simulink model "DDR_KinematicModel"  (R2019b)
settings: Solver=FixedStepAuto  StartTime=0.0  StopTime=10  FixedStep=0.001  RelTol=1e-3
undefined symbols (not defined in the file): a, phi_init, v0, x_init, xi, y_init
libraries: simulink x1
settings Model: Creator=DanielleNasrallah  LastModifiedBy=kerrm
settings DataIOCC: ReturnWorkspaceOutputs=off

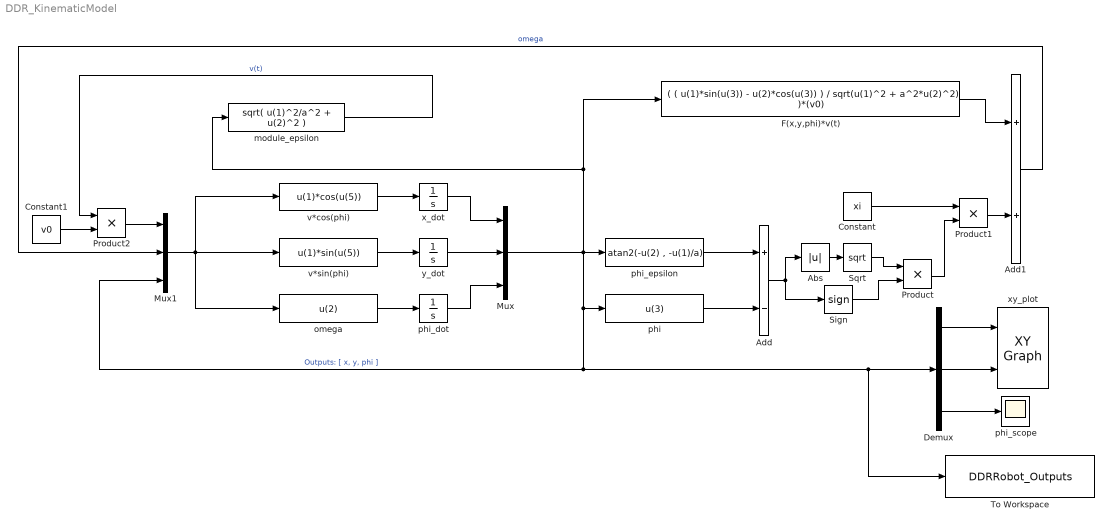
== system DDR_KinematicModel ==
  Abs : Abs
  Add : Sum  Inputs=+-
  Add1 : Sum
  Constant : Constant  Value=xi
  Constant1 : Constant  Value=v0
  Demux : Demux  Outputs=3
  F(x,y,phi)*v(t) : Fcn  Expr=( ( u(1)*sin(u(3)) - u(2)*cos(u(3)) ) / sqrt(u(1)^2 + a^2*u(2)^2) )*(v0)
  Mux : Mux  Inputs=3
  Mux1 : Mux  Inputs=3
  Product : Product
  Product1 : Product
  Product2 : Product
  Sign : Signum
  Sqrt : Sqrt  SaturateOnIntegerOverflow=on
  To Workspace : ToWorkspace  VariableName=DDRRobot_Outputs  SampleTime=-1
      settings: Save2DSignal=2-D array (concatenate along first dimension)
  "module_epsilon " : Fcn  Expr=sqrt( u(1)^2/a^2 + u(2)^2 )
  "omega " : Fcn  Expr=u(2)
  phi : Fcn  Expr=u(3)
  phi_dot : Integrator  InitialCondition=phi_init
  phi_epsilon : Fcn  Expr=atan2(-u(2) , -u(1)/a)
  phi_scope : Scope
  v*cos(phi) : Fcn  Expr=u(1)*cos(u(5))
  v*sin(phi) : Fcn  Expr=u(1)*sin(u(5))
  x_dot : Integrator  InitialCondition=x_init
  xy_plot : simulink/Sinks/XY Graph  xmin=-5  xmax=5  ymin=-5  ymax=5  st=-1
  y_dot : Integrator  InitialCondition=y_init
  wires:
  y_dot/1 -> Mux/2
  x_dot/1 -> Mux/1
  phi_dot/1 -> Mux/3
  Mux1/1 -> v*cos(phi)/1, "omega "/1, v*sin(phi)/1
  v*cos(phi)/1 -> x_dot/1
  v*sin(phi)/1 -> y_dot/1
  "omega "/1 -> phi_dot/1
  phi_epsilon/1 -> Add/1
  phi/1 -> Add/2
  Add1/1 -> Mux1/2  "omega"
  Demux/2 -> xy_plot/2
  Demux/1 -> xy_plot/1
  Mux/1 -> Mux1/3, To Workspace/1, Demux/1, phi/1, phi_epsilon/1, "module_epsilon "/1, F(x,y,phi)*v(t)/1  "Outputs: [ x, y, phi ]"
  Demux/3 -> phi_scope/1
  Add/1 -> Abs/1, Sign/1
  Abs/1 -> Sqrt/1
  Sqrt/1 -> Product/1
  Sign/1 -> Product/2
  Product/1 -> Product1/2
  "module_epsilon "/1 -> Product2/1  "v(t)"
  Product1/1 -> Add1/2
  F(x,y,phi)*v(t)/1 -> Add1/1
  Product2/1 -> Mux1/1
  Constant1/1 -> Product2/2
  Constant/1 -> Product1/1
